simulink model "ukol_6_model"  (R2017a)
settings: Solver=VariableStepAuto  StartTime=0.0  StopTime=10  RelTol=1e-3
libraries: cstblocks x2
settings Model: Creator=tomas  LastModifiedBy=tomas

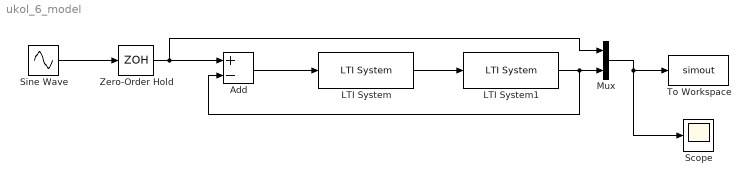
== system ukol_6_model ==
  Add : Sum  Inputs=+-
  LTI System : cstblocks/LTI System  sys=Fr_6  IC=[]
  LTI System1 : cstblocks/LTI System  sys=discrete_Fs  IC=[]
  Mux : Mux  Inputs=2
  Scope : Scope
  Sine Wave : Sin  SampleTime=0
  To Workspace : ToWorkspace  VariableName=simout  SaveFormat=Timeseries  SampleTime=-1
  Zero-Order Hold : ZeroOrderHold  SampleTime=0.2
  wires:
  Sine Wave/1 -> Zero-Order Hold/1
  Add/1 -> LTI System/1
  LTI System/1 -> LTI System1/1
  Mux/1 -> Scope/1, To Workspace/1
  LTI System1/1 -> Add/2, Mux/2
  Zero-Order Hold/1 -> Mux/1, Add/1
